simulink model "PWMGenerator_v3"  (R2016b)
settings: Solver=VariableStepAuto  StartTime=0.0  StopTime=10.0  RelTol=1e-3
settings Model: Creator=paul.rogers  LastModifiedBy=paul.rogers
settings OptimizationCC: BlockReduction=off  ConditionallyExecuteInputs=off  DefaultParameterBehavior=Inlined
settings DebuggingCC: AlgebraicLoopMsg=error
settings HardwareCC: ProdBitPerPointer=32  ProdBitPerSizeT=32  ProdBitPerPtrDiffT=32  ProdLargestAtomicFloat=None  ProdIntDivRoundTo=Undefined  ProdEndianess=Unspecified  ProdWordSize=32  ProdHWDeviceType=ASIC/FPGA->ASIC/FPGA  ProdEqTarget=off

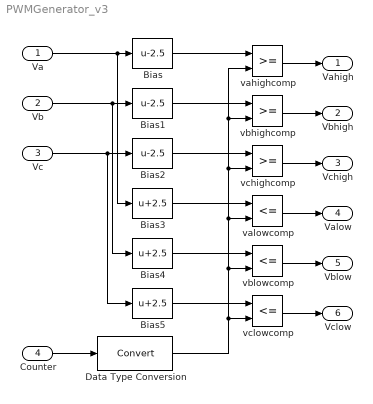
== system PWMGenerator_v3 ==
  Va : Inport  OutDataTypeStr=fixdt(1,84,66)  SampleTime=2e-6
  Vb : Inport  Port=2  OutDataTypeStr=fixdt(1,84,66)  SampleTime=2e-6
  Vc : Inport  Port=3  OutDataTypeStr=fixdt(1,84,66)  SampleTime=2e-6
  Counter : Inport  Port=4  OutDataTypeStr=uint8  SampleTime=2e-6
  Bias : Bias  Bias=-2.5
  Bias1 : Bias  Bias=-2.5
  Bias2 : Bias  Bias=-2.5
  Bias3 : Bias  Bias=2.5
  Bias4 : Bias  Bias=2.5
  Bias5 : Bias  Bias=2.5
  Data Type Conversion : DataTypeConversion
  vahighcomp : RelationalOperator  RndMeth=Nearest
  valowcomp : RelationalOperator  Operator=<=  RndMeth=Nearest
  vbhighcomp : RelationalOperator  RndMeth=Nearest
  vblowcomp : RelationalOperator  Operator=<=  RndMeth=Nearest
  vchighcomp : RelationalOperator  RndMeth=Nearest
  vclowcomp : RelationalOperator  Operator=<=  RndMeth=Nearest
  Vahigh : Outport
  Vbhigh : Outport  Port=2
  Vchigh : Outport  Port=3
  Valow : Outport  Port=4
  Vblow : Outport  Port=5
  Vclow : Outport  Port=6
  wires:
  vahighcomp/1 -> Vahigh/1
  vclowcomp/1 -> Vclow/1
  vbhighcomp/1 -> Vbhigh/1
  vblowcomp/1 -> Vblow/1
  vchighcomp/1 -> Vchigh/1
  valowcomp/1 -> Valow/1
  Data Type Conversion/1 -> vblowcomp/2, valowcomp/2, vahighcomp/2, vbhighcomp/2, vchighcomp/2, vclowcomp/2
  Counter/1 -> Data Type Conversion/1
  Va/1 -> Bias3/1, Bias/1
  Vb/1 -> Bias4/1, Bias1/1
  Vc/1 -> Bias5/1, Bias2/1
  Bias5/1 -> vclowcomp/1
  Bias4/1 -> vblowcomp/1
  Bias3/1 -> valowcomp/1
  Bias2/1 -> vchighcomp/1
  Bias1/1 -> vbhighcomp/1
  Bias/1 -> vahighcomp/1
